simulink model "exercise03"  (R2022a)
settings: Solver=VariableStepAuto  StartTime=0.0  StopTime=10.0  RelTol=1e-3
PostLoadFcn:
  | if exist('09_Entwurfsverfahren', 'dir')
  | addpath('09_Entwurfsverfahren')
  | end
libraries: simulink x1
settings Model: Creator=ac133867  LastModifiedBy=cunis
settings DebuggingCC: UnconnectedInputMsg=warning  UnconnectedOutputMsg=warning  UnconnectedLineMsg=warning
settings RTWCC: DLArmComputeVersion=19.05

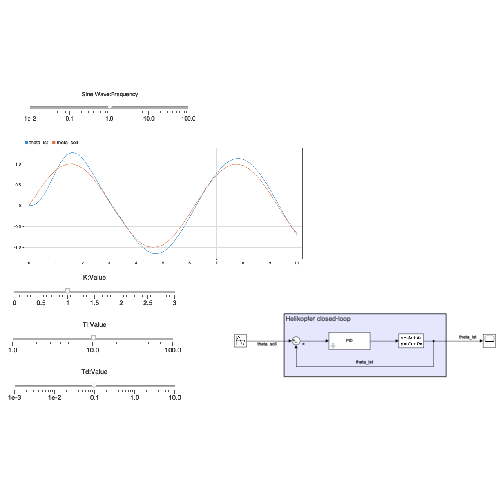
[thumbnail: Simulink's stored preview of the top-level diagram]
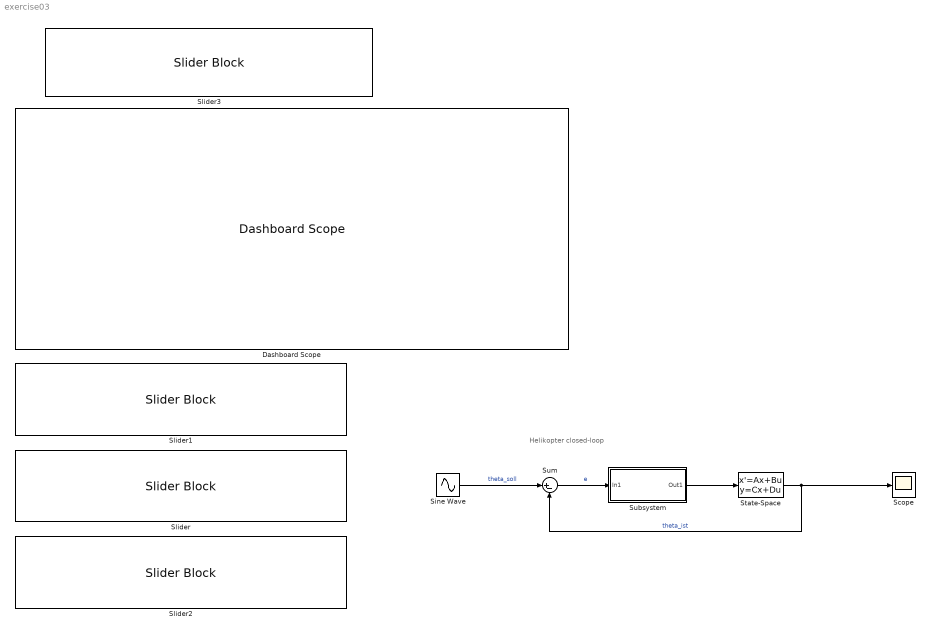
== system exercise03 ==
  note: Helikopter closed-loop
  Dashboard Scope : DashboardScope
  Scope : Scope
  Sine Wave : Sin  Frequency=1.015339550826043  SampleTime=0
  Slider : SliderBlock  ScaleMin=1  ScaleType=Log
  Slider1 : SliderBlock  ScaleMax=3  TickInterval=0.5
  Slider2 : SliderBlock  ScaleMin=0.001  ScaleMax=10  ScaleType=Log
  Slider3 : SliderBlock  ScaleMin=0.01  ScaleType=Log
  State-Space : StateSpace  A=[-0.2040 1.392 -9.8019; 0.0073 -0.4875 -0.0313; 0 1 0]  B=[-2.1242; 8.2631;0]  C=[0;0;1]'  D=0  InitialCondition=0
  Subsystem : Subsystem
      mask Display: disp('PID');
  Sum : Sum  Inputs=|+-
  wires:
  Sine Wave/1 -> Sum/1  "theta_soll"
  State-Space/1 -> Scope/1, Sum/2  "theta_ist"
  Sum/1 -> Subsystem/1(In1)  "e"
  Subsystem/1(Out1) -> State-Space/1

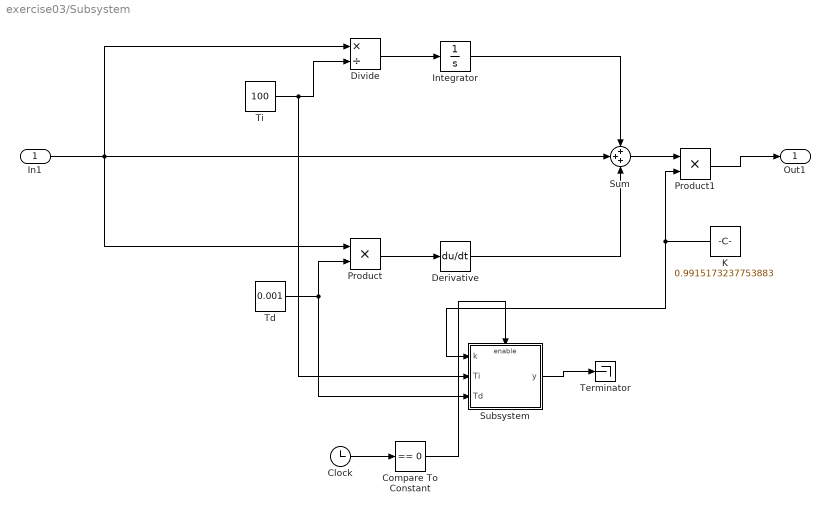
== system exercise03/Subsystem ==
  In1 : Inport
  Clock : Clock
  Compare To Constant : simulink/Logic and Bit Operations/Compare To Constant  relop===  const=0  OutDataTypeStr=boolean
  Derivative : Derivative
  Divide : Product  Inputs=*/
  Integrator : Integrator
  K : Constant  Value=0.9915173237753883
  Product : Product
  Product1 : Product
  Subsystem : Subsystem
  Sum : Sum  Inputs=+++
  Td : Constant  Value=0.001
  Terminator : Terminator
  Ti : Constant  Value=100
  Out1 : Outport
  wires:
  Sum/1 -> Product1/1
  In1/1 -> Product/1, Divide/1, Sum/2
  Integrator/1 -> Sum/1
  Divide/1 -> Integrator/1
  Ti/1 -> Subsystem/2(Ti), Divide/2
  Product1/1 -> Out1/1
  K/1 -> Subsystem/1(k), Product1/2
  Td/1 -> Subsystem/3(Td), Product/2
  Product/1 -> Derivative/1
  Derivative/1 -> Sum/3
  Subsystem/1(y) -> Terminator/1
  Clock/1 -> Compare To Constant/1
  Compare To Constant/1 -> Subsystem/Enable

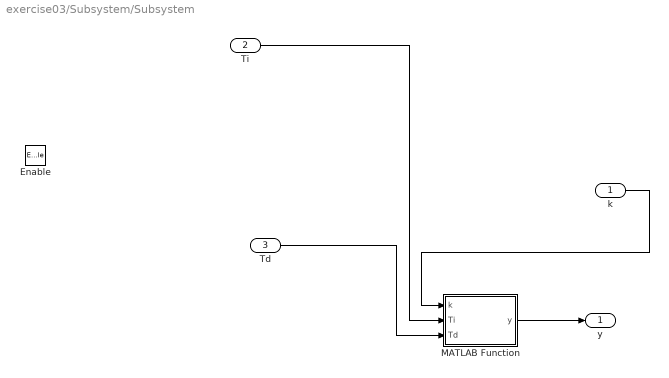
== system exercise03/Subsystem/Subsystem ==
  k : Inport
  Ti : Inport  Port=2
  Td : Inport  Port=3
  Enable : EnablePort
  MATLAB Function : MATLAB Function  TreatAsAtomicUnit=on
  y : Outport
  wires:
  k/1 -> MATLAB Function/1(k)
  Ti/1 -> MATLAB Function/2(Ti)
  Td/1 -> MATLAB Function/3(Td)
  MATLAB Function/1(y) -> y/1

== matlab function exercise03/Subsystem/Subsystem/MATLAB Function ==
  data: k input; y output; Ti input; Td input
function y = fcn(k,Ti,Td)

coder.extrinsic('bodeplot');

bodeplot(k,Ti,Td);

y = 0;

end
